simulink model "Create4x4matrix"  (Simulink 7.4)
settings: Solver=ode45  StartTime=0.0  StopTime=10.0  RelTol=1e-3
values from neighbouring files (symbols this model uses):
  K_pitch = 0.8    [PID_init.m]
  K_roll = 0.8    [PID_init.m]
  K_yaw = 0.8    [PID_init.m]
  Ti_pitch = 0.000    (= 0)    [PID_init.m]
  Ti_roll = 0.000    (= 0)    [PID_init.m]
  Ti_yaw = 0.000    (= 0)    [PID_init.m]
settings Model: Creator=diogo  LastModifiedBy=diogo

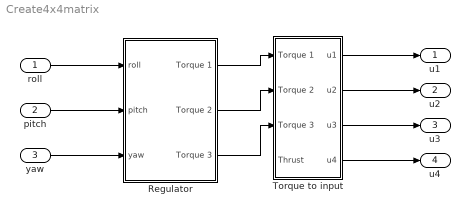
== system Create4x4matrix ==
  roll : Inport  OutDataType=fixdt(1, 16)  OutScaling=2^0
  pitch : Inport  Port=2  OutDataType=fixdt(1, 16)  OutScaling=2^0
  yaw : Inport  Port=3  OutDataType=fixdt(1, 16)  OutScaling=2^0
  Regulator : Subsystem
  Torque to input : Subsystem
  " u1" : Outport  OutDataType=fixdt(1, 16)  OutScaling=2^0
  " u2" : Outport  Port=2  OutDataType=fixdt(1, 16)  OutScaling=2^0
  " u3" : Outport  Port=3  OutDataType=fixdt(1, 16)  OutScaling=2^0
  " u4" : Outport  Port=4  OutDataType=fixdt(1, 16)  OutScaling=2^0
  wires:
  roll/1 -> Regulator/1(roll)
  pitch/1 -> Regulator/2(pitch)
  yaw/1 -> Regulator/3(yaw)
  Torque to input/1(" u1") -> " u1"/1
  Torque to input/2(" u2") -> " u2"/1
  Torque to input/3(" u3") -> " u3"/1
  Torque to input/4(" u4") -> " u4"/1
  Regulator/1(" Torque 1") -> Torque to input/1(Torque 1)
  Regulator/2(" Torque 2") -> Torque to input/2(Torque 2)
  Regulator/3(" Torque 3") -> Torque to input/3(Torque 3)

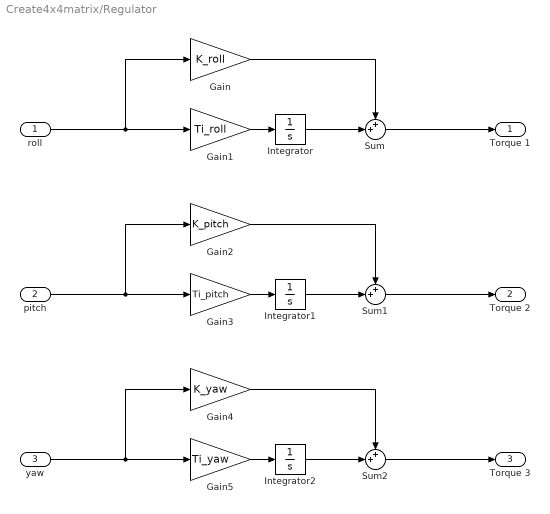
== system Create4x4matrix/Regulator ==
  roll : Inport  OutDataType=fixdt(1, 16)  OutScaling=2^0
  pitch : Inport  Port=2  OutDataType=fixdt(1, 16)  OutScaling=2^0
  yaw : Inport  Port=3  OutDataType=fixdt(1, 16)  OutScaling=2^0
  Gain : Gain  Gain=K_roll  ParameterDataType=fixdt(1, 16)  ParameterScaling=2^0  OutDataType=fixdt(1, 16)  OutScaling=2^0
  Gain1 : Gain  Gain=Ti_roll  ParameterDataType=fixdt(1, 16)  ParameterScaling=2^0  OutDataType=fixdt(1, 16)  OutScaling=2^0
  Gain2 : Gain  Gain=K_pitch  ParameterDataType=fixdt(1, 16)  ParameterScaling=2^0  OutDataType=fixdt(1, 16)  OutScaling=2^0
  Gain3 : Gain  Gain=Ti_pitch  ParameterDataType=fixdt(1, 16)  ParameterScaling=2^0  OutDataType=fixdt(1, 16)  OutScaling=2^0
  Gain4 : Gain  Gain=K_yaw  ParameterDataType=fixdt(1, 16)  ParameterScaling=2^0  OutDataType=fixdt(1, 16)  OutScaling=2^0
  Gain5 : Gain  Gain=Ti_yaw  ParameterDataType=fixdt(1, 16)  ParameterScaling=2^0  OutDataType=fixdt(1, 16)  OutScaling=2^0
  Integrator : Integrator
  Integrator1 : Integrator
  Integrator2 : Integrator
  Sum : Sum  Inputs=++|  OutDataType=fixdt(1, 16)  OutScaling=2^0
  Sum1 : Sum  Inputs=++|  OutDataType=fixdt(1, 16)  OutScaling=2^0
  Sum2 : Sum  Inputs=++|  OutDataType=fixdt(1, 16)  OutScaling=2^0
  " Torque 1" : Outport  OutDataType=fixdt(1, 16)  OutScaling=2^0
  " Torque 2" : Outport  Port=2  OutDataType=fixdt(1, 16)  OutScaling=2^0
  " Torque 3" : Outport  Port=3  OutDataType=fixdt(1, 16)  OutScaling=2^0
  wires:
  roll/1 -> Gain1/1, Gain/1
  Gain/1 -> Sum/1
  Gain1/1 -> Integrator/1
  Integrator/1 -> Sum/2
  Sum/1 -> " Torque 1"/1
  pitch/1 -> Gain3/1, Gain2/1
  Gain2/1 -> Sum1/1
  Gain3/1 -> Integrator1/1
  Integrator1/1 -> Sum1/2
  yaw/1 -> Gain5/1, Gain4/1
  Gain4/1 -> Sum2/1
  Gain5/1 -> Integrator2/1
  Integrator2/1 -> Sum2/2
  Sum1/1 -> " Torque 2"/1
  Sum2/1 -> " Torque 3"/1

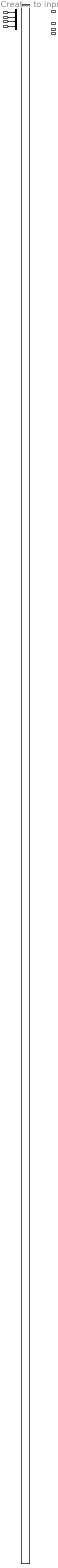
== system Create4x4matrix/Torque to input ==
  Torque 1 : Inport  OutDataType=fixdt(1, 16)  OutScaling=2^0
  Torque 2 : Inport  Port=2  OutDataType=fixdt(1, 16)  OutScaling=2^0
  Torque 3 : Inport  Port=3  OutDataType=fixdt(1, 16)  OutScaling=2^0
  Thrust : Inport  Port=4  OutDataType=fixdt(1, 16)  OutScaling=2^0
  Create 3x3 Matrix1 : Subsystem  AncestorBlock=aerolibutil/Create 3x3 Matrix  mask(Create 3x3 Matrix){}
      mask help:
      | Create a 3-by-3 matrix from nine input values. Each input corresponds to an element of the matrix.
      |
      | For example, the input labeled A21 is the entry in the second row and first column of the matrix.
      mask init:
      | aeroicon('aeroblk');
      mask Help: eval('asbhelp(''create_threebythree_matrix'')');
      mask Display:
      | port_label('input',1,'A_{11}','texmode','on');
      | port_label('input',2,'A_{12}','texmode','on');
      | port_label('input',3,'A_{13}','texmode','on');
      | port_label('input',4,'A_{21}','texmode','on');
      | port_label('input',5,'A_{22}','texmode','on');
      | port_label('input',6,'A_{23}','texmode','on');
      | port_label('input',7,'A_{31}','texmode','on');
      | port_label('input',8,'A_{32}','texmode','on');
      | port_label('input',9,'A_{33}','texmode','on');
      | port_label('output',1,'A','texmode','on');
  Mux : Mux
  " u1" : Outport  OutDataType=fixdt(1, 16)  OutScaling=2^0
  " u2" : Outport  Port=2  OutDataType=fixdt(1, 16)  OutScaling=2^0
  " u3" : Outport  Port=3  OutDataType=fixdt(1, 16)  OutScaling=2^0
  " u4" : Outport  Port=4  OutDataType=fixdt(1, 16)  OutScaling=2^0
  wires:
  Thrust/1 -> Mux/1
  Torque 1/1 -> Mux/2
  Torque 2/1 -> Mux/3
  Torque 3/1 -> Mux/4

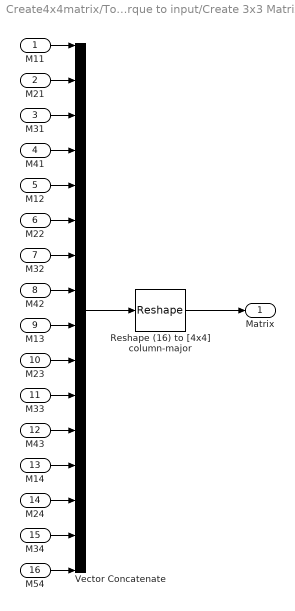
== system Create4x4matrix/Torque to input/Create 3x3 Matrix1 ==
  M11 : Inport  PortDimensions=1  OutDataType=sfix(16)  OutScaling=2^0
  M21 : Inport  Port=2  PortDimensions=1  OutDataType=sfix(16)  OutScaling=2^0
  M31 : Inport  Port=3  PortDimensions=1  OutDataType=sfix(16)  OutScaling=2^0
  M41 : Inport  Port=4  PortDimensions=1  OutDataType=sfix(16)  OutScaling=2^0
  M12 : Inport  Port=5  PortDimensions=1  OutDataType=sfix(16)  OutScaling=2^0
  M22 : Inport  Port=6  PortDimensions=1  OutDataType=sfix(16)  OutScaling=2^0
  M32 : Inport  Port=7  PortDimensions=1  OutDataType=sfix(16)  OutScaling=2^0
  M42 : Inport  Port=8  PortDimensions=1  OutDataType=sfix(16)  OutScaling=2^0
  M13 : Inport  Port=9  PortDimensions=1  OutDataType=sfix(16)  OutScaling=2^0
  M23 : Inport  Port=10  PortDimensions=1  OutDataType=sfix(16)  OutScaling=2^0
  M33 : Inport  Port=11  PortDimensions=1  OutDataType=sfix(16)  OutScaling=2^0
  M43 : Inport  Port=12  PortDimensions=1  OutDataType=sfix(16)  OutScaling=2^0
  M14 : Inport  Port=13  PortDimensions=1  OutDataType=sfix(16)  OutScaling=2^0
  M24 : Inport  Port=14  PortDimensions=1  OutDataType=sfix(16)  OutScaling=2^0
  M34 : Inport  Port=15  PortDimensions=1  OutDataType=sfix(16)  OutScaling=2^0
  M54 : Inport  Port=16  PortDimensions=1  OutDataType=sfix(16)  OutScaling=2^0
  Reshape (16) to [4x4] column-major : Reshape  OutputDimensionality=Customize  OutputDimensions=[4,4]
  Vector Concatenate : Concatenate  NumInputs=16  Mode=Vector
  Matrix : Outport  PortDimensions=[3 3]  OutDataType=sfix(16)  OutScaling=2^0
  wires:
  Vector Concatenate/1 -> Reshape (16) to [4x4] column-major/1
  M11/1 -> Vector Concatenate/1
  M21/1 -> Vector Concatenate/2
  M31/1 -> Vector Concatenate/3
  M41/1 -> Vector Concatenate/4
  M12/1 -> Vector Concatenate/5
  Reshape (16) to [4x4] column-major/1 -> Matrix/1
  M13/1 -> Vector Concatenate/9
  M22/1 -> Vector Concatenate/6
  M32/1 -> Vector Concatenate/7
  M23/1 -> Vector Concatenate/10
  M33/1 -> Vector Concatenate/11
  M42/1 -> Vector Concatenate/8
  M43/1 -> Vector Concatenate/12
  M14/1 -> Vector Concatenate/13
  M24/1 -> Vector Concatenate/14
  M34/1 -> Vector Concatenate/15
  M54/1 -> Vector Concatenate/16
